simulink model "VDSE_2019b1"  (R2022b)
settings: Solver=ode5  StartTime=0.0  StopTime=T_simulation  FixedStep=simulation_step_time  RelTol=1e-3
values from neighbouring files (symbols this model uses):
  A = 2    [vehicle_parameters_script.m]
  bump_height = 0    [vehicle_parameters_script.m]
  bump_length = 0    [vehicle_parameters_script.m]
  bump_time = 0    [vehicle_parameters_script.m]
  cd = 0.35    [vehicle_parameters_script.m]
  cF = 5000    [vehicle_parameters_script.m]
  clF = -0.15    [vehicle_parameters_script.m]
  clR = -0.20    (= -0.2)    [vehicle_parameters_script.m]
  cp_FA = 30    [vehicle_parameters_script.m]
  cp_RA = 13    [vehicle_parameters_script.m]
  cR = 5000    [vehicle_parameters_script.m]
  ctF = tireF.VERTICAL_DAMPING    [vehicle_parameters_script.m]
  ctR = tireR.VERTICAL_DAMPING    [vehicle_parameters_script.m]
  enableDriverControl = 1    [vehicle_parameters_script.m]
  enableLongDynamics = 1    [vehicle_parameters_script.m]
  enablePowertrain = 1    [vehicle_parameters_script.m]
  g = 9.806    [vehicle_parameters_script.m]
  Gear_numbers = [1 2 3 4 5 6]    [vehicle_parameters_script.m]
  GR = [2.9 1.8 1.3 1 0.85 0.75]    [vehicle_parameters_script.m]
  hcog = 0.441    [vehicle_parameters_script.m]
  hpc = 0.0    (= 0)    [vehicle_parameters_script.m]
  hrcF = 0.3    [vehicle_parameters_script.m]
  hrcg = (hrcF*lR+hrcR*lF)/(lF+lR)    (= 0.25108)    [vehicle_parameters_script.m]
  hrcR = 0.2    [vehicle_parameters_script.m]
  huFcog = 0.32    [vehicle_parameters_script.m]
  huRcog = 0.32    [vehicle_parameters_script.m]
  i1 = 11.42    [vehicle_parameters_script.m]
  i2 = 3.727    [vehicle_parameters_script.m]
  initial_gear = 1    [vehicle_parameters_script.m]
  JwF = 2.45    [vehicle_parameters_script.m]
  JwR = 2.45    [vehicle_parameters_script.m]
  Jx = 4.12    [vehicle_parameters_script.m]
  Jy = 109.16    [vehicle_parameters_script.m]
  Jz = 105.13    [vehicle_parameters_script.m]
  kF = 40000    [vehicle_parameters_script.m]
  kR = 35000    [vehicle_parameters_script.m]
  kRF = 0    [vehicle_parameters_script.m]
  kRR = 0    [vehicle_parameters_script.m]
  ktF = tireF.VERTICAL_STIFFNESS    [vehicle_parameters_script.m]
  ktR = tireR.VERTICAL_STIFFNESS    [vehicle_parameters_script.m]
  lF = 1.223    [vehicle_parameters_script.m]
  lR = l-lF    (= 1.277)    [vehicle_parameters_script.m]
  m = 340    [vehicle_parameters_script.m]
  max_pressure = 1000    [vehicle_parameters_script.m]
  maxrpm = 4000    [vehicle_parameters_script.m]
  mF = 45    [vehicle_parameters_script.m]
  minrpm = 1500    [vehicle_parameters_script.m]
  mR = 50    [vehicle_parameters_script.m]
  output_samping_time = 0.001    [vehicle_parameters_script.m]
  phi0 = 0    [vehicle_parameters_script.m]
  phi_dot0 = 0    [vehicle_parameters_script.m]
  psi0 = 0    [vehicle_parameters_script.m]
  psi_dot0 = 0    [vehicle_parameters_script.m]
  RearRatio = 1    [vehicle_parameters_script.m]
  requested_speed = 120/3.6    (= 33.3333333333)    [vehicle_parameters_script.m]
  rF = tireF.UNLOADED_RADIUS    [vehicle_parameters_script.m]
  rho = 1.2    [vehicle_parameters_script.m]
  rR = tireR.UNLOADED_RADIUS    [vehicle_parameters_script.m]
  steer_ratio = 13.25    [vehicle_parameters_script.m]
  TFL = 0    [vehicle_parameters_script.m]
  TFR = 0    [vehicle_parameters_script.m]
  theta0 = 0    [vehicle_parameters_script.m]
  theta_dot0 = 0    [vehicle_parameters_script.m]
  TRL = 0    [vehicle_parameters_script.m]
  TRR = 0    [vehicle_parameters_script.m]
  Vx0 = 0.01/3.6    (= 0.00277777777778)    [vehicle_parameters_script.m]
  Vy0 = 0    [vehicle_parameters_script.m]
  Vz0 = 0    [vehicle_parameters_script.m]
  wF = 1.578    [vehicle_parameters_script.m]
  wR = 1.544    [vehicle_parameters_script.m]
  x0 = 0    [vehicle_parameters_script.m]
  xcog_overall = (2*mR*xR+2*xF*mF+m*xs)/(m+2*mF+2*mR)    (= 1.25626415094)    [vehicle_parameters_script.m]
  y0 = 0    [vehicle_parameters_script.m]
  z0 = 0    [vehicle_parameters_script.m]
  zFL0 = 0    [vehicle_parameters_script.m]
  zFL_dot0 = 0    [vehicle_parameters_script.m]
  zFR0 = 0    [vehicle_parameters_script.m]
  zFR_dot0 = 0    [vehicle_parameters_script.m]
  zRL0 = 0    [vehicle_parameters_script.m]
  zRL_dot0 = 0    [vehicle_parameters_script.m]
  zRR0 = 0    [vehicle_parameters_script.m]
  zRR_dot0 = 0    [vehicle_parameters_script.m]
undefined symbols (not defined in the file or in its folder): Bxf, Bxr, Byf, Byr, Cxf, Cxr, Cyf, Cyr, DiscIntNeverNeededParam, Dxf, Dxr, Dyf, Dyr, exf, exr, eyf, eyr, FNOMINf, FNOMINr, Ldwf, Ldwr, PCX1f, PCX1r, PCY1f, PCY1r, PDX1f, PDX1r, PDX2f, PDX2r, PDY1f, PDY1r, PDY2f, PDY2r, PDY3f, PDY3r, PEX1f, PEX1r, PEX2f, PEX2r, PEX3f, PEX3r, PEX4f, PEX4r, PEY1f, PEY1r, PEY2f, PEY2r, PEY3f, PEY3r, PEY4f, PEY4r, PHX1f, PHX1r, PHX2f, PHX2r, PHY1f, PHY1r, PHY2f, PHY2r, PHY3f ... (+147)
libraries: simulink x55, mfeval_LIB x4, slpidlib x1
(part 4 of 7)

== system VDSE_2019b1/14-DOF VEHICLE MODEL/SUSPENSION/FRONT SUSPENSION/SUSPENSION FL ==
  z [m] : Inport
  Vz [m/s] : Inport  Port=2
  phi [rad] : Inport  Port=3
  phi_dot [rad/s] : Inport  Port=4
  theta [rad] : Inport  Port=5
  theta_dot [rad/s] : Inport  Port=6
  zFR [m] : Inport  Port=7
  yFL_road [m] : Inport  Port=8
  FL : Subsystem
  TIRE VERTICAL DEFLECTION : Subsystem
  fFLz [N] : Outport
  zFL_dot [m/s] : Outport  Port=2
  zFL [m] : Outport  Port=3
  wires:
  FL/2(zFL_dot [m/s]) -> TIRE VERTICAL DEFLECTION/2(zFL_dot [m/s]), zFL_dot [m/s]/1
  z [m]/1 -> FL/1(z [m])
  TIRE VERTICAL DEFLECTION/1(fFLz [N]) -> fFLz [N]/1
  theta [rad]/1 -> FL/5(theta [rad])
  zFR [m]/1 -> FL/7(zFR [m])
  Vz [m/s]/1 -> FL/2(Vz [m/s])
  yFL_road [m]/1 -> TIRE VERTICAL DEFLECTION/3(yFL_road [m]), FL/8(yFL_road [m])
  phi_dot [rad/s]/1 -> FL/4(phi_dot [rad/s])
  FL/1(zFL [m]) -> TIRE VERTICAL DEFLECTION/1(zFL [m]), zFL [m]/1
  phi [rad]/1 -> FL/3(phi [rad])
  theta_dot [rad/s]/1 -> FL/6(theta_dot [rad/s])

== system VDSE_2019b1/14-DOF VEHICLE MODEL/SUSPENSION/FRONT SUSPENSION/SUSPENSION FR ==
  z [m] : Inport
  Vz [m/s] : Inport  Port=2
  phi [rad] : Inport  Port=3
  phi_dot [rad/s] : Inport  Port=4
  theta [rad] : Inport  Port=5
  theta_dot [rad/s] : Inport  Port=6
  zFL [m] : Inport  Port=7
  yFR_road [m] : Inport  Port=8
  FR : Subsystem
  TIRE VERTICAL DEFLECTION : Subsystem
  fFRz [N] : Outport
  zFR [m] : Outport  Port=2
  zFR_dot [m/s] : Outport  Port=3
  wires:
  FR/2(zFR_dot [m/s]) -> zFR_dot [m/s]/1, TIRE VERTICAL DEFLECTION/2(zFR_dot [m/s])
  yFR_road [m]/1 -> FR/8(yFR_road [m]), TIRE VERTICAL DEFLECTION/3(yFR_road [m])
  z [m]/1 -> FR/1(z [m])
  TIRE VERTICAL DEFLECTION/1(fFRz [N]) -> fFRz [N]/1
  theta [rad]/1 -> FR/5(theta [rad])
  zFL [m]/1 -> FR/7(zFL [m])
  Vz [m/s]/1 -> FR/2(Vz [m/s])
  phi_dot [rad/s]/1 -> FR/4(phi_dot [rad/s])
  FR/1(zFR [m]) -> TIRE VERTICAL DEFLECTION/1(zFR [m]), zFR [m]/1
  phi [rad]/1 -> FR/3(phi [rad])
  theta_dot [rad/s]/1 -> FR/6(theta_dot [rad/s])

== system VDSE_2019b1/14-DOF VEHICLE MODEL/SUSPENSION/Load Transfer/Coupling of load transfer and suspension reaction ==
  Longidutinal Load Transfer [N] : Inport
  Lateral Load Transfer - Front [N] : Inport  Port=2
  Lateral Load Transfer - Rear [N] : Inport  Port=3
  <fFLz [N]> : Inport  Port=4
  <fFRz [N]> : Inport  Port=5
  <fRLz [N]> : Inport  Port=6
  <fRRz [N]> : Inport  Port=7
  Add{,1..4} (5 alike) : Sum
  Add5 : Sum  Inputs=+-
  Add6 : Sum  Inputs=-+
  Add7 : Sum  Inputs=--
  Lateral Load Transfer - Front [N]1 : InportShadow  Port=2
  Lateral Load Transfer - Rear [N]1 : InportShadow  Port=3
  Longidutinal Load Transfer [N]1 : InportShadow
  Longidutinal Load Transfer [N]2 : InportShadow
  Longidutinal Load Transfer [N]3 : InportShadow
  FLz_Overall [N] : Outport
  FRz_Overall [N] : Outport  Port=2
  RLz_Overall [N] : Outport  Port=3
  RRz_Overall [N] : Outport  Port=4
  wires:
  <fFRz [N]>/1 -> Add1/2
  Lateral Load Transfer - Rear [N]/1 -> Add5/2
  Longidutinal Load Transfer [N]/1 -> Add7/1
  Add7/1 -> Add/1  "FL Dynamic LT"
  Lateral Load Transfer - Front [N]/1 -> Add7/2
  Add4/1 -> Add3/1  "RR Dynamic LT"
  Add6/1 -> Add1/1  "FR Dynamic LT"
  Add5/1 -> Add2/1  "RL Dynamic LT"
  <fRRz [N]>/1 -> Add3/2
  <fFLz [N]>/1 -> Add/2
  <fRLz [N]>/1 -> Add2/2
  Add1/1 -> FRz_Overall [N]/1  "FRz_Overall [N]"
  Add3/1 -> RRz_Overall [N]/1  "RRz_Overall [N]"
  Add/1 -> FLz_Overall [N]/1  "FLz_Overall [N]"
  Add2/1 -> RLz_Overall [N]/1  "RLz_Overall [N]"
  Longidutinal Load Transfer [N]1/1 -> Add6/1
  Longidutinal Load Transfer [N]2/1 -> Add5/1
  Longidutinal Load Transfer [N]3/1 -> Add4/1
  Lateral Load Transfer - Front [N]1/1 -> Add6/2
  Lateral Load Transfer - Rear [N]1/1 -> Add4/2

== system VDSE_2019b1/14-DOF VEHICLE MODEL/SUSPENSION/Load Transfer/Dynamic Lateral Load Transfer - Front ==
  ay [m/s^2] : Inport
  Add : Sum
  Gain : Gain  Gain=lR/(lR+lF)
  Gain1 : Gain  Gain=2*mF*huFcog/wF
  Gain2 : Gain  Gain=m*hrcF/wF
  Lat. Dynamic Transfer [N] : Outport
  wires:
  ay [m/s^2]/1 -> Gain2/1, Gain1/1
  Gain2/1 -> Gain/1
  Add/1 -> Lat. Dynamic Transfer [N]/1
  Gain1/1 -> Add/2
  Gain/1 -> Add/1

== system VDSE_2019b1/14-DOF VEHICLE MODEL/SUSPENSION/Load Transfer/Dynamic Lateral Load Transfer - Rear ==
  ay [m/s^2] : Inport
  Add : Sum
  Gain : Gain  Gain=lF/(lR+lF)
  Gain1 : Gain  Gain=2*mR*huRcog/wR
  Gain2 : Gain  Gain=m*hrcR/wR
  Lat. Dynamic Transfer [N] : Outport
  wires:
  Add/1 -> Lat. Dynamic Transfer [N]/1
  Gain1/1 -> Add/2
  ay [m/s^2]/1 -> Gain2/1, Gain1/1
  Gain2/1 -> Gain/1
  Gain/1 -> Add/1

== system VDSE_2019b1/14-DOF VEHICLE MODEL/SUSPENSION/Load Transfer/Dynamic Longitudinal Load Transfer ==
  ax [m/s^2] : Inport
  Add : Sum
  Gain : Gain  Gain=1/2*hpc*m/(lF+lR)/2
  Gain1 : Gain  Gain=(mF*huFcog + mR*huRcog)/(lF+lR)
  Long. Dynamic Transfer [N] : Outport
  wires:
  ax [m/s^2]/1 -> Gain1/1, Gain/1
  Gain/1 -> Add/1
  Add/1 -> Long. Dynamic Transfer [N]/1
  Gain1/1 -> Add/2

== system VDSE_2019b1/14-DOF VEHICLE MODEL/SUSPENSION/REAR SUSPENSION/SUSPENSION RL ==
  z [m] : Inport
  Vz [m/s] : Inport  Port=2
  phi [rad] : Inport  Port=3
  phi_dot [rad/s] : Inport  Port=4
  theta [rad] : Inport  Port=5
  theta_dot [rad/s] : Inport  Port=6
  zRR [m] : Inport  Port=7
  yRL_road [m] : Inport  Port=8
  RL : Subsystem
  TIRE VERTICAL DEFLECTION : Subsystem
  fRLz [N] : Outport
  zRL_dot [m/s] : Outport  Port=2
  zRL [m] : Outport  Port=3
  wires:
  RL/2(zRL_dot [m/s]) -> TIRE VERTICAL DEFLECTION/2(zRL_dot [m/s]), zRL_dot [m/s]/1
  z [m]/1 -> RL/1(z [m])
  TIRE VERTICAL DEFLECTION/1(fRLz [N]) -> fRLz [N]/1  "fRLz [N]"
  theta [rad]/1 -> RL/5(theta [rad])
  zRR [m]/1 -> RL/7(zRR [m])
  Vz [m/s]/1 -> RL/2(Vz [m/s])
  yRL_road [m]/1 -> TIRE VERTICAL DEFLECTION/3(yRL_road [m]), RL/8(yRL_road [m])
  phi_dot [rad/s]/1 -> RL/4(phi_dot [rad/s])
  RL/1(zRL [m]) -> TIRE VERTICAL DEFLECTION/1(zRL [m]), zRL [m]/1
  phi [rad]/1 -> RL/3(phi [rad])
  theta_dot [rad/s]/1 -> RL/6(theta_dot [rad/s])

== system VDSE_2019b1/14-DOF VEHICLE MODEL/SUSPENSION/REAR SUSPENSION/SUSPENSION RR ==
  z [m] : Inport
  Vz [m/s] : Inport  Port=2
  phi [rad] : Inport  Port=3
  phi_dot [rad/s] : Inport  Port=4
  theta [rad] : Inport  Port=5
  theta_dot [rad/s] : Inport  Port=6
  zRL [m] : Inport  Port=7
  yRR_road [m] : Inport  Port=8
  RR : Subsystem
  TIRE VERTICAL DEFLECTION : Subsystem
  fRRz [N] : Outport
  zRR [m] : Outport  Port=2
  zRR_dot [m/s] : Outport  Port=3
  wires:
  RR/2(zRR_dot [m/s]) -> TIRE VERTICAL DEFLECTION/2(zRR_dot [m/s]), zRR_dot [m/s]/1
  yRR_road [m]/1 -> TIRE VERTICAL DEFLECTION/3(yRR_road [m]), RR/8(yRR_road [m])
  z [m]/1 -> RR/1(z [m])
  TIRE VERTICAL DEFLECTION/1(fRRz [N]) -> fRRz [N]/1
  theta [rad]/1 -> RR/5(theta [rad])
  zRL [m]/1 -> RR/7(zRL [m])
  Vz [m/s]/1 -> RR/2(Vz [m/s])
  phi_dot [rad/s]/1 -> RR/4(phi_dot [rad/s])
  RR/1(zRR [m]) -> TIRE VERTICAL DEFLECTION/1(zRR [m]), zRR [m]/1
  phi [rad]/1 -> RR/3(phi [rad])
  theta_dot [rad/s]/1 -> RR/6(theta_dot [rad/s])

== system VDSE_2019b1/14-DOF VEHICLE MODEL/WHEEL ASSEMBLY/WHEEL ASSEMBLY BCD/SIDE SLIP ANGLE CALCULATION ==
  Vx [m/s] : Inport
  Vy [m/s] : Inport  Port=2
  Add : Sum
  Atan2 : Trigonometry  Operator=atan2
  Clock : Clock
  Constant : Constant  Value=enableLongDynamics
  Constant1 : Constant  Value=Vx0
  Constant2 : Constant  Value=0
  Sqrt : Sqrt
  Square : Math  Operator=square
  Square1 : Math  Operator=square
  Switch : Switch  Criteria=u2 > Threshold  SaturateOnIntegerOverflow=off  InputSameDT=off
  Switch1 : Switch  Criteria=u2 > Threshold  Threshold=0.01  SaturateOnIntegerOverflow=off  InputSameDT=off
  Vy [m/s]1 : InportShadow  Port=2
  V [m/s] : Outport
  beta [rad] : Outport  Port=2
  wires:
  Clock/1 -> Switch1/2
  Constant2/1 -> Switch1/3
  Switch1/1 -> Switch/2
  Constant1/1 -> Switch/3
  Constant/1 -> Switch1/1
  Switch/1 -> Atan2/2, Square/1
  Square1/1 -> Add/2
  Square/1 -> Add/1
  Vy [m/s]/1 -> Square1/1
  Vx [m/s]/1 -> Switch/1
  Add/1 -> Sqrt/1
  Sqrt/1 -> V [m/s]/1
  Atan2/1 -> beta [rad]/1
  Vy [m/s]1/1 -> Atan2/1

== system VDSE_2019b1/14-DOF VEHICLE MODEL/WHEEL ASSEMBLY/WHEEL ASSEMBLY BCD/TIRE PARAMETERS ==
  Constant : Constant  Value=Bxf
  Constant1 : Constant  Value=Cxf
  Constant10 : Constant  Value=Cyr
  Constant11 : Constant  Value=Dyr
  Constant2 : Constant  Value=Dxf
  Constant3 : Constant  Value=Bxr
  Constant4 : Constant  Value=Cxr
  Constant5 : Constant  Value=Dxr
  Constant6 : Constant  Value=Byf
  Constant7 : Constant  Value=Cyf
  Constant8 : Constant  Value=Dyf
  Constant9 : Constant  Value=Byr
  Bxf : Outport
  Cxf : Outport  Port=2
  Dxf : Outport  Port=3
  Bxr : Outport  Port=4
  Cxr : Outport  Port=5
  Dxr : Outport  Port=6
  Byf : Outport  Port=7
  Cyf : Outport  Port=8
  Dyf : Outport  Port=9
  Byr : Outport  Port=10
  Cyr : Outport  Port=11
  Dyr : Outport  Port=12
  wires:
  Constant/1 -> Bxf/1
  Constant1/1 -> Cxf/1
  Constant2/1 -> Dxf/1
  Constant5/1 -> Dxr/1
  Constant4/1 -> Cxr/1
  Constant3/1 -> Bxr/1
  Constant9/1 -> Byr/1
  Constant10/1 -> Cyr/1
  Constant11/1 -> Dyr/1
  Constant8/1 -> Dyf/1
  Constant7/1 -> Cyf/1
  Constant6/1 -> Byf/1

== system VDSE_2019b1/14-DOF VEHICLE MODEL/WHEEL ASSEMBLY/WHEEL ASSEMBLY MFEVAL/SIDE SLIP ANGLE CALCULATION ==
  Vx [m/s] : Inport
  Vy [m/s] : Inport  Port=2
  Add : Sum
  Atan2 : Trigonometry  Operator=atan2
  Clock : Clock
  Constant : Constant  Value=enableLongDynamics
  Constant1 : Constant  Value=Vx0
  Constant2 : Constant  Value=0
  Sqrt : Sqrt
  Square : Math  Operator=square
  Square1 : Math  Operator=square
  Switch : Switch  Criteria=u2 > Threshold  SaturateOnIntegerOverflow=off  InputSameDT=off
  Switch1 : Switch  Criteria=u2 > Threshold  Threshold=0.01  SaturateOnIntegerOverflow=off  InputSameDT=off
  Vy [m/s]1 : InportShadow  Port=2
  V [m/s] : Outport
  beta [rad] : Outport  Port=2
  wires:
  Clock/1 -> Switch1/2
  Constant2/1 -> Switch1/3
  Switch1/1 -> Switch/2
  Constant1/1 -> Switch/3
  Constant/1 -> Switch1/1
  Square1/1 -> Add/2
  Square/1 -> Add/1
  Vy [m/s]/1 -> Square1/1
  Vx [m/s]/1 -> Switch/1
  Add/1 -> Sqrt/1
  Atan2/1 -> beta [rad]/1
  Vy [m/s]1/1 -> Atan2/1
  Switch/1 -> Atan2/2, Square/1
  Sqrt/1 -> V [m/s]/1

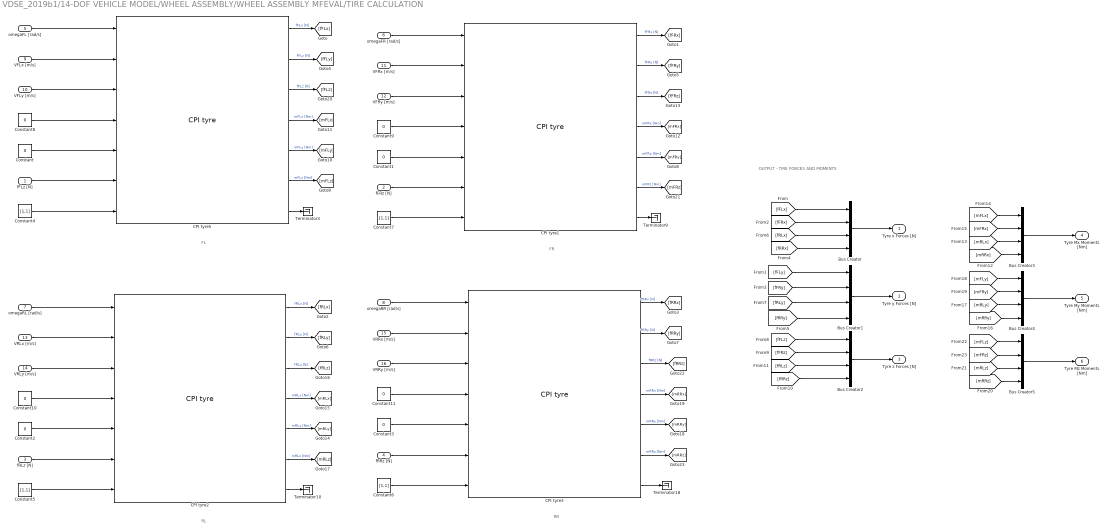
== system VDSE_2019b1/14-DOF VEHICLE MODEL/WHEEL ASSEMBLY/WHEEL ASSEMBLY MFEVAL/TIRE CALCULATION ==
  note: RR
  note: RL
  note: FR
  note: FL
  note: OUTPUT - TIRE FORCES AND MOMENTS
  fFLz [N] : Inport
  fFRz [N] : Inport  Port=2
  fRLz [N] : Inport  Port=3
  fRRz [N] : Inport  Port=4
  omegaFL [rad/s] : Inport  Port=5
  omegaFR [rad/s] : Inport  Port=6
  omegaRL [rad/s] : Inport  Port=7
  omegaRR [rad/s] : Inport  Port=8
  VFLx [m/s] : Inport  Port=9
  VFLy [m/s] : Inport  Port=10
  VFRx [m/s] : Inport  Port=11
  VFRy [m/s] : Inport  Port=12
  VRLx [m/s] : Inport  Port=13
  VRLy [m/s] : Inport  Port=14
  VRRx [m/s] : Inport  Port=15
  VRRy [m/s] : Inport  Port=16
  Bus Creator{,1..5} (6 alike) : BusCreator  Inputs=4
  CPI tyre1 : mfeval_LIB/CPI tyre  Description=Magic Formula 6.1.2 tyre model including relaxation length and transient calculations  userParameterSource=tir_file_front  userSide=2 right  userDynamics=1 steady state  userUseMode=1 combined  enablePressure=off  userPressure=2.3
      settings: SourceProductName=MFeval Library
  CPI tyre2 : mfeval_LIB/CPI tyre  Description=Magic Formula 6.1.2 tyre model including relaxation length and transient calculations  userParameterSource=tir_file_rear  userSide=1 left  userDynamics=1 steady state  userUseMode=1 combined  enablePressure=off  userPressure=2.3
      settings: SourceProductName=MFeval Library
  CPI tyre3 : mfeval_LIB/CPI tyre  Description=Magic Formula 6.1.2 tyre model including relaxation length and transient calculations  userParameterSource=tir_file_rear  userSide=2 right  userDynamics=1 steady state  userUseMode=1 combined  enablePressure=off  userPressure=2.3
      settings: SourceProductName=MFeval Library
  CPI tyre5 : mfeval_LIB/CPI tyre  Description=Magic Formula 6.1.2 tyre model including relaxation length and transient calculations  userParameterSource=tir_file_front  userSide=1 left  userDynamics=1 steady state  userUseMode=1 combined  enablePressure=off  userPressure=2.3
      settings: SourceProductName=MFeval Library
  Constant{,1..3,8..11} (8 alike) : Constant  Value=0
  Constant{4..7} (4 alike) : Constant  Value=[1,1]
  Terminator{3,9..10,18} (4 alike) : Terminator
  Tyre x Forces [N] : Outport
  Tyre y Forces [N] : Outport  Port=2
  Tyre z Forces [N] : Outport  Port=3
  Tyre Mx Moments [Nm] : Outport  Port=4
  Tyre My Moments [Nm] : Outport  Port=5
  Tyre Mz Moments [Nm] : Outport  Port=6
  wires:
  Constant11/1 -> CPI tyre3/4
  Constant10/1 -> CPI tyre2/4
  Constant9/1 -> CPI tyre1/4
  Constant8/1 -> CPI tyre5/4
  CPI tyre3/3 -> [fRRz]  "fRRz [N]"
  CPI tyre3/6 -> [mRRz]  "mRRz [Nm]"
  CPI tyre3/4 -> [mRRx]  "mRRx [Nm]"
  CPI tyre3/5 -> [mRRy]  "mRRy [Nm]"
  CPI tyre2/3 -> [fRLz]  "fRLz [N]"
  CPI tyre2/6 -> [mRLz]  "mRLz [Nm]"
  CPI tyre2/4 -> [mRLx]  "mRLx [Nm]"
  CPI tyre2/5 -> [mRLy]  "mRLy [Nm]"
  CPI tyre1/3 -> [fFRz]  "fFRz [N]"
  CPI tyre1/6 -> [mFRz]  "mFRz [Nm]"
  CPI tyre1/4 -> [mFRx]  "mFRx [Nm]"
  CPI tyre1/5 -> [mFRy]  "mFRy [Nm]"
  CPI tyre5/3 -> [fFLz]  "fFLz [N]"
  CPI tyre5/4 -> [mFLx]  "mFLx [Nm]"
  CPI tyre5/5 -> [mFLy]  "mFLy [Nm]"
  Bus Creator5/1 -> Tyre Mz Moments [Nm]/1
  [mFRz] -> Bus Creator5/2
  [mRLz] -> Bus Creator5/3
  [mRRz] -> Bus Creator5/4
  [mFLz] -> Bus Creator5/1
  [mFLy] -> Bus Creator4/1
  [mRRy] -> Bus Creator4/4
  [mRLy] -> Bus Creator4/3
  [mFRy] -> Bus Creator4/2
  Bus Creator4/1 -> Tyre My Moments [Nm]/1
  Bus Creator3/1 -> Tyre Mx Moments [Nm]/1
  [mFRx] -> Bus Creator3/2
  [mRLx] -> Bus Creator3/3
  [mRRx] -> Bus Creator3/4
  [mFLx] -> Bus Creator3/1
  [fFLz] -> Bus Creator2/1
  [fRRz] -> Bus Creator2/4
  [fRLz] -> Bus Creator2/3
  [fFRz] -> Bus Creator2/2
  Bus Creator2/1 -> Tyre z Forces [N]/1
  Bus Creator1/1 -> Tyre y Forces [N]/1
  Bus Creator/1 -> Tyre x Forces [N]/1
  [fFRy] -> Bus Creator1/2
  [fRLy] -> Bus Creator1/3
  [fRRy] -> Bus Creator1/4
  [fFLy] -> Bus Creator1/1
  [fRRx] -> Bus Creator/4
  [fRLx] -> Bus Creator/3
  [fFRx] -> Bus Creator/2
  [fFLx] -> Bus Creator/1
  CPI tyre3/2 -> [fRRy]  "fRRy [N]"
  CPI tyre2/2 -> [fRLy]  "fRLy [N]"
  CPI tyre1/2 -> [fFRy]  "fFRy [N]"
  CPI tyre5/2 -> [fFLy]  "fFLy [N]"
  CPI tyre2/1 -> [fRLx]  "fRLx [N]"
  CPI tyre3/1 -> [fRRx]  "fRRx [N]"
  CPI tyre1/1 -> [fFRx]  "fFRx [N]"
  CPI tyre5/1 -> [fFLx]  "fFLx [N]"
  CPI tyre3/7 -> Terminator18/1
  CPI tyre2/7 -> Terminator10/1
  CPI tyre1/7 -> Terminator9/1
  CPI tyre5/7 -> Terminator3/1
  CPI tyre5/6 -> [mFLz]  "mFLz [Nm]"
  VRRx [m/s]/1 -> CPI tyre3/2
  VRRy [m/s]/1 -> CPI tyre3/3
  VRLy [m/s]/1 -> CPI tyre2/3
  VRLx [m/s]/1 -> CPI tyre2/2
  VFRy [m/s]/1 -> CPI tyre1/3
  VFRx [m/s]/1 -> CPI tyre1/2
  VFLx [m/s]/1 -> CPI tyre5/2
  VFLy [m/s]/1 -> CPI tyre5/3
  omegaRR [rad/s]/1 -> CPI tyre3/1
  omegaRL [rad/s]/1 -> CPI tyre2/1
  omegaFR [rad/s]/1 -> CPI tyre1/1
  omegaFL [rad/s]/1 -> CPI tyre5/1
  Constant7/1 -> CPI tyre1/7
  Constant6/1 -> CPI tyre3/7
  Constant5/1 -> CPI tyre2/7
  Constant4/1 -> CPI tyre5/7
  Constant3/1 -> CPI tyre3/5
  Constant2/1 -> CPI tyre2/5
  Constant1/1 -> CPI tyre1/5
  Constant/1 -> CPI tyre5/5
  fFLz [N]/1 -> CPI tyre5/6
  fRLz [N]/1 -> CPI tyre2/6
  fRRz [N]/1 -> CPI tyre3/6
  fFRz [N]/1 -> CPI tyre1/6

== system VDSE_2019b1/14-DOF VEHICLE MODEL/WHEEL ASSEMBLY/WHEEL ASSEMBLY PACEIJKA/SIDE SLIP ANGLE CALCULATION ==
  Vx [m/s] : Inport
  Vy [m/s] : Inport  Port=2
  Add : Sum
  Atan2 : Trigonometry  Operator=atan2
  Clock : Clock
  Constant : Constant  Value=enableLongDynamics
  Constant1 : Constant  Value=Vx0
  Constant2 : Constant  Value=0
  Sqrt : Sqrt
  Square : Math  Operator=square
  Square1 : Math  Operator=square
  Switch : Switch  Criteria=u2 > Threshold  SaturateOnIntegerOverflow=off  InputSameDT=off
  Switch1 : Switch  Criteria=u2 > Threshold  Threshold=0.01  SaturateOnIntegerOverflow=off  InputSameDT=off
  Vy [m/s]1 : InportShadow  Port=2
  V [m/s] : Outport
  beta [rad] : Outport  Port=2
  wires:
  Vy [m/s]1/1 -> Atan2/1
  Atan2/1 -> beta [rad]/1
  Sqrt/1 -> V [m/s]/1
  Add/1 -> Sqrt/1
  Vx [m/s]/1 -> Switch/1
  Vy [m/s]/1 -> Square1/1
  Square/1 -> Add/1
  Square1/1 -> Add/2
  Switch/1 -> Atan2/2, Square/1
  Constant/1 -> Switch1/1
  Constant1/1 -> Switch/3
  Switch1/1 -> Switch/2
  Constant2/1 -> Switch1/3
  Clock/1 -> Switch1/2

== system VDSE_2019b1/14-DOF VEHICLE MODEL/WHEEL ASSEMBLY/WHEEL ASSEMBLY PACEIJKA/TIRE PARAMETERS ==
  Mux1 : Mux  Inputs=91
  Mux2 : Mux  Inputs=91
  TIRE PARAMETERS - FRONT AXLE : Subsystem
  TIRE PARAMETERS - REAR AXLE : Subsystem
  Tire Parameters Front Axle : Outport
  Tire Parameters Rear Axle : Outport  Port=2
  wires:
  TIRE PARAMETERS - FRONT AXLE/29(PCY1) -> Mux1/29
  TIRE PARAMETERS - FRONT AXLE/18(PKY3) -> Mux1/18
  TIRE PARAMETERS - FRONT AXLE/1(PHX1) -> Mux1/1
  TIRE PARAMETERS - FRONT AXLE/48(RVY4) -> Mux1/48
  TIRE PARAMETERS - FRONT AXLE/41(RBY1) -> Mux1/41
  TIRE PARAMETERS - FRONT AXLE/8(PEX3) -> Mux1/8
  TIRE PARAMETERS - FRONT AXLE/23(PHY1) -> Mux1/23
  TIRE PARAMETERS - FRONT AXLE/46(RVY2) -> Mux1/46
  TIRE PARAMETERS - FRONT AXLE/5(PCX1) -> Mux1/5
  TIRE PARAMETERS - FRONT AXLE/19(PVY1) -> Mux1/19
  TIRE PARAMETERS - FRONT AXLE/22(PVY4) -> Mux1/22
  TIRE PARAMETERS - FRONT AXLE/53(RHY1) -> Mux1/53
  TIRE PARAMETERS - FRONT AXLE/7(PEX2) -> Mux1/7
  TIRE PARAMETERS - FRONT AXLE/37(RCX1) -> Mux1/37
  TIRE PARAMETERS - FRONT AXLE/51(REY1) -> Mux1/51
  TIRE PARAMETERS - FRONT AXLE/28(PDY3) -> Mux1/28
  TIRE PARAMETERS - FRONT AXLE/36(RBX2) -> Mux1/36
  TIRE PARAMETERS - FRONT AXLE/34(ey) -> Mux1/34
  TIRE PARAMETERS - FRONT AXLE/10(PKX1) -> Mux1/10
  TIRE PARAMETERS - FRONT AXLE/30(PEY1) -> Mux1/30
  TIRE PARAMETERS - FRONT AXLE/17(PKY2) -> Mux1/17
  TIRE PARAMETERS - FRONT AXLE/2(PHX2) -> Mux1/2
  TIRE PARAMETERS - FRONT AXLE/33(PEY4) -> Mux1/33
  TIRE PARAMETERS - FRONT AXLE/39(REX2) -> Mux1/39
  TIRE PARAMETERS - FRONT AXLE/45(RVY1) -> Mux1/45
  TIRE PARAMETERS - FRONT AXLE/52(REY2) -> Mux1/52
  TIRE PARAMETERS - FRONT AXLE/21(PVY3) -> Mux1/21
  TIRE PARAMETERS - FRONT AXLE/3(PDX1) -> Mux1/3
  TIRE PARAMETERS - FRONT AXLE/6(PEX1) -> Mux1/6
  TIRE PARAMETERS - FRONT AXLE/4(PDX2) -> Mux1/4
  TIRE PARAMETERS - FRONT AXLE/49(RVY5) -> Mux1/49
  TIRE PARAMETERS - FRONT AXLE/44(RCY1) -> Mux1/44
  TIRE PARAMETERS - FRONT AXLE/25(PHY3) -> Mux1/25
  TIRE PARAMETERS - FRONT AXLE/24(PHY2) -> Mux1/24
  TIRE PARAMETERS - FRONT AXLE/54(RHY2) -> Mux1/54
  TIRE PARAMETERS - FRONT AXLE/43(RBY3) -> Mux1/43
  TIRE PARAMETERS - FRONT AXLE/13(ex) -> Mux1/13
  TIRE PARAMETERS - FRONT AXLE/31(PEY2) -> Mux1/31
  TIRE PARAMETERS - FRONT AXLE/14(PVX1) -> Mux1/14
  TIRE PARAMETERS - FRONT AXLE/35(RBX1) -> Mux1/35
  TIRE PARAMETERS - FRONT AXLE/15(PVX2) -> Mux1/15
  TIRE PARAMETERS - FRONT AXLE/27(PDY2) -> Mux1/27
  TIRE PARAMETERS - FRONT AXLE/20(PVY2) -> Mux1/20
  TIRE PARAMETERS - FRONT AXLE/11(PKX2) -> Mux1/11
  TIRE PARAMETERS - FRONT AXLE/50(RVY6) -> Mux1/50
  TIRE PARAMETERS - FRONT AXLE/32(PEY3) -> Mux1/32
  Mux1/1 -> Tire Parameters Front Axle/1
  TIRE PARAMETERS - FRONT AXLE/47(RVY3) -> Mux1/47
  TIRE PARAMETERS - FRONT AXLE/9(PEX4) -> Mux1/9
  TIRE PARAMETERS - FRONT AXLE/40(RHX1) -> Mux1/40
  TIRE PARAMETERS - FRONT AXLE/38(REX1) -> Mux1/38
  TIRE PARAMETERS - FRONT AXLE/42(RBY2) -> Mux1/42
  TIRE PARAMETERS - FRONT AXLE/26(PDY1) -> Mux1/26
  TIRE PARAMETERS - FRONT AXLE/12(PKX3) -> Mux1/12
  TIRE PARAMETERS - FRONT AXLE/16(PKY1) -> Mux1/16
  TIRE PARAMETERS - REAR AXLE/16(PKY1) -> Mux2/16
  TIRE PARAMETERS - REAR AXLE/12(PKX3) -> Mux2/12
  TIRE PARAMETERS - REAR AXLE/26(PDY1) -> Mux2/26
  TIRE PARAMETERS - REAR AXLE/42(RBY2) -> Mux2/42
  TIRE PARAMETERS - REAR AXLE/38(REX1) -> Mux2/38
  TIRE PARAMETERS - REAR AXLE/40(RHX1) -> Mux2/40
  TIRE PARAMETERS - REAR AXLE/9(PEX4) -> Mux2/9
  TIRE PARAMETERS - REAR AXLE/47(RVY3) -> Mux2/47
  Mux2/1 -> Tire Parameters Rear Axle/1
  TIRE PARAMETERS - REAR AXLE/32(PEY3) -> Mux2/32
  TIRE PARAMETERS - REAR AXLE/50(RVY6) -> Mux2/50
  TIRE PARAMETERS - REAR AXLE/11(PKX2) -> Mux2/11
  TIRE PARAMETERS - REAR AXLE/20(PVY2) -> Mux2/20
  TIRE PARAMETERS - REAR AXLE/27(PDY2) -> Mux2/27
  TIRE PARAMETERS - REAR AXLE/15(PVX2) -> Mux2/15
  TIRE PARAMETERS - REAR AXLE/35(RBX1) -> Mux2/35
  TIRE PARAMETERS - REAR AXLE/14(PVX1) -> Mux2/14
  TIRE PARAMETERS - REAR AXLE/31(PEY2) -> Mux2/31
  TIRE PARAMETERS - REAR AXLE/13(ex) -> Mux2/13
  TIRE PARAMETERS - REAR AXLE/43(RBY3) -> Mux2/43
  TIRE PARAMETERS - REAR AXLE/54(RHY2) -> Mux2/54
  TIRE PARAMETERS - REAR AXLE/24(PHY2) -> Mux2/24
  TIRE PARAMETERS - REAR AXLE/25(PHY3) -> Mux2/25
  TIRE PARAMETERS - REAR AXLE/44(RCY1) -> Mux2/44
  TIRE PARAMETERS - REAR AXLE/49(RVY5) -> Mux2/49
  TIRE PARAMETERS - REAR AXLE/4(PDX2) -> Mux2/4
  TIRE PARAMETERS - REAR AXLE/6(PEX1) -> Mux2/6
  TIRE PARAMETERS - REAR AXLE/3(PDX1) -> Mux2/3
  TIRE PARAMETERS - REAR AXLE/21(PVY3) -> Mux2/21
  TIRE PARAMETERS - REAR AXLE/52(REY2) -> Mux2/52
  TIRE PARAMETERS - REAR AXLE/45(RVY1) -> Mux2/45
  TIRE PARAMETERS - REAR AXLE/39(REX2) -> Mux2/39
  TIRE PARAMETERS - REAR AXLE/33(PEY4) -> Mux2/33
  TIRE PARAMETERS - REAR AXLE/2(PHX2) -> Mux2/2
  TIRE PARAMETERS - REAR AXLE/17(PKY2) -> Mux2/17
  TIRE PARAMETERS - REAR AXLE/30(PEY1) -> Mux2/30
  TIRE PARAMETERS - REAR AXLE/10(PKX1) -> Mux2/10
  TIRE PARAMETERS - REAR AXLE/34(ey) -> Mux2/34
  TIRE PARAMETERS - REAR AXLE/36(RBX2) -> Mux2/36
  TIRE PARAMETERS - REAR AXLE/28(PDY3) -> Mux2/28
  TIRE PARAMETERS - REAR AXLE/51(REY1) -> Mux2/51
  TIRE PARAMETERS - REAR AXLE/37(RCX1) -> Mux2/37
  TIRE PARAMETERS - REAR AXLE/7(PEX2) -> Mux2/7
  TIRE PARAMETERS - REAR AXLE/53(RHY1) -> Mux2/53
  TIRE PARAMETERS - REAR AXLE/22(PVY4) -> Mux2/22
  TIRE PARAMETERS - REAR AXLE/19(PVY1) -> Mux2/19
  TIRE PARAMETERS - REAR AXLE/5(PCX1) -> Mux2/5
  TIRE PARAMETERS - REAR AXLE/46(RVY2) -> Mux2/46
  TIRE PARAMETERS - REAR AXLE/23(PHY1) -> Mux2/23
  TIRE PARAMETERS - REAR AXLE/8(PEX3) -> Mux2/8
  TIRE PARAMETERS - REAR AXLE/41(RBY1) -> Mux2/41
  TIRE PARAMETERS - REAR AXLE/48(RVY4) -> Mux2/48
  TIRE PARAMETERS - REAR AXLE/1(PHX1) -> Mux2/1
  TIRE PARAMETERS - REAR AXLE/18(PKY3) -> Mux2/18
  TIRE PARAMETERS - REAR AXLE/29(PCY1) -> Mux2/29
  TIRE PARAMETERS - REAR AXLE/55(FNOMIN) -> Mux2/55
  TIRE PARAMETERS - FRONT AXLE/55(FNOMIN) -> Mux1/55
  TIRE PARAMETERS - FRONT AXLE/56(QHZ1) -> Mux1/56
  TIRE PARAMETERS - FRONT AXLE/57(QHZ2) -> Mux1/57
  TIRE PARAMETERS - FRONT AXLE/58(QHZ3) -> Mux1/58
  TIRE PARAMETERS - FRONT AXLE/59(QHZ4) -> Mux1/59
  TIRE PARAMETERS - FRONT AXLE/60(QBZ1) -> Mux1/60
  TIRE PARAMETERS - FRONT AXLE/61(QBZ2) -> Mux1/61
  TIRE PARAMETERS - FRONT AXLE/62(QBZ3) -> Mux1/62
  TIRE PARAMETERS - FRONT AXLE/63(QBZ4) -> Mux1/63
  TIRE PARAMETERS - FRONT AXLE/64(QBZ5) -> Mux1/64
  TIRE PARAMETERS - FRONT AXLE/65(QCZ1) -> Mux1/65
  TIRE PARAMETERS - FRONT AXLE/66(QDZ1) -> Mux1/66
  TIRE PARAMETERS - FRONT AXLE/67(QDZ2) -> Mux1/67
  TIRE PARAMETERS - FRONT AXLE/68(QDZ3) -> Mux1/68
  TIRE PARAMETERS - FRONT AXLE/69(QDZ4) -> Mux1/69
  TIRE PARAMETERS - FRONT AXLE/70(QEZ1) -> Mux1/70
  TIRE PARAMETERS - FRONT AXLE/71(QEZ2) -> Mux1/71
  TIRE PARAMETERS - FRONT AXLE/72(QEZ3) -> Mux1/72
  TIRE PARAMETERS - FRONT AXLE/73(QEZ4) -> Mux1/73
  TIRE PARAMETERS - FRONT AXLE/74(QEZ5) -> Mux1/74
  TIRE PARAMETERS - FRONT AXLE/75(QBZ9) -> Mux1/75
  TIRE PARAMETERS - FRONT AXLE/76(QBZ10) -> Mux1/76
  TIRE PARAMETERS - FRONT AXLE/77(QDZ6) -> Mux1/77
  TIRE PARAMETERS - FRONT AXLE/78(QDZ7) -> Mux1/78
  TIRE PARAMETERS - FRONT AXLE/79(QDZ8) -> Mux1/79
  TIRE PARAMETERS - FRONT AXLE/80(QDZ9) -> Mux1/80
  TIRE PARAMETERS - FRONT AXLE/81(R0) -> Mux1/81
  TIRE PARAMETERS - FRONT AXLE/82(zeta7) -> Mux1/82
  TIRE PARAMETERS - FRONT AXLE/83(SSZ1) -> Mux1/83
  TIRE PARAMETERS - FRONT AXLE/84(SSZ2) -> Mux1/84
  TIRE PARAMETERS - FRONT AXLE/85(SSZ3) -> Mux1/85
  TIRE PARAMETERS - FRONT AXLE/86(SSZ4) -> Mux1/86
  TIRE PARAMETERS - FRONT AXLE/87(QSY1) -> Mux1/87
  TIRE PARAMETERS - FRONT AXLE/88(QSY2) -> Mux1/88
  TIRE PARAMETERS - FRONT AXLE/89(QSY3) -> Mux1/89
  TIRE PARAMETERS - FRONT AXLE/90(QSY4) -> Mux1/90
  TIRE PARAMETERS - FRONT AXLE/91(VREF) -> Mux1/91
  TIRE PARAMETERS - REAR AXLE/56(QHZ1) -> Mux2/56
  TIRE PARAMETERS - REAR AXLE/57(QHZ2) -> Mux2/57
  TIRE PARAMETERS - REAR AXLE/58(QHZ3) -> Mux2/58
  TIRE PARAMETERS - REAR AXLE/59(QHZ4) -> Mux2/59
  TIRE PARAMETERS - REAR AXLE/60(QBZ1) -> Mux2/60
  TIRE PARAMETERS - REAR AXLE/61(QBZ2) -> Mux2/61
  TIRE PARAMETERS - REAR AXLE/62(QBZ3) -> Mux2/62
  TIRE PARAMETERS - REAR AXLE/63(QBZ4) -> Mux2/63
  TIRE PARAMETERS - REAR AXLE/64(QBZ5) -> Mux2/64
  TIRE PARAMETERS - REAR AXLE/65(QCZ1) -> Mux2/65
  TIRE PARAMETERS - REAR AXLE/66(QDZ1) -> Mux2/66
  TIRE PARAMETERS - REAR AXLE/67(QDZ2) -> Mux2/67
  TIRE PARAMETERS - REAR AXLE/68(QDZ3) -> Mux2/68
  TIRE PARAMETERS - REAR AXLE/69(QDZ4) -> Mux2/69
  TIRE PARAMETERS - REAR AXLE/70(QEZ1) -> Mux2/70
  TIRE PARAMETERS - REAR AXLE/71(QEZ2) -> Mux2/71
  TIRE PARAMETERS - REAR AXLE/72(QEZ3) -> Mux2/72
  TIRE PARAMETERS - REAR AXLE/73(QEZ4) -> Mux2/73
  TIRE PARAMETERS - REAR AXLE/74(QEZ5) -> Mux2/74
  TIRE PARAMETERS - REAR AXLE/75(QBZ9) -> Mux2/75
  TIRE PARAMETERS - REAR AXLE/76(QBZ10) -> Mux2/76
  TIRE PARAMETERS - REAR AXLE/77(QDZ6) -> Mux2/77
  TIRE PARAMETERS - REAR AXLE/78(QDZ7) -> Mux2/78
  TIRE PARAMETERS - REAR AXLE/79(QDZ8) -> Mux2/79
  TIRE PARAMETERS - REAR AXLE/80(QDZ9) -> Mux2/80
  TIRE PARAMETERS - REAR AXLE/81(R0) -> Mux2/81
  TIRE PARAMETERS - REAR AXLE/82(zeta7) -> Mux2/82
  TIRE PARAMETERS - REAR AXLE/83(SSZ1) -> Mux2/83
  TIRE PARAMETERS - REAR AXLE/84(SSZ2) -> Mux2/84
  TIRE PARAMETERS - REAR AXLE/85(SSZ3) -> Mux2/85
  TIRE PARAMETERS - REAR AXLE/86(SSZ4) -> Mux2/86
  TIRE PARAMETERS - REAR AXLE/87(QSY1) -> Mux2/87
  TIRE PARAMETERS - REAR AXLE/88(QSY2) -> Mux2/88
  TIRE PARAMETERS - REAR AXLE/89(QSY3) -> Mux2/89
  TIRE PARAMETERS - REAR AXLE/90(QSY4) -> Mux2/90
  TIRE PARAMETERS - REAR AXLE/91(VREF) -> Mux2/91

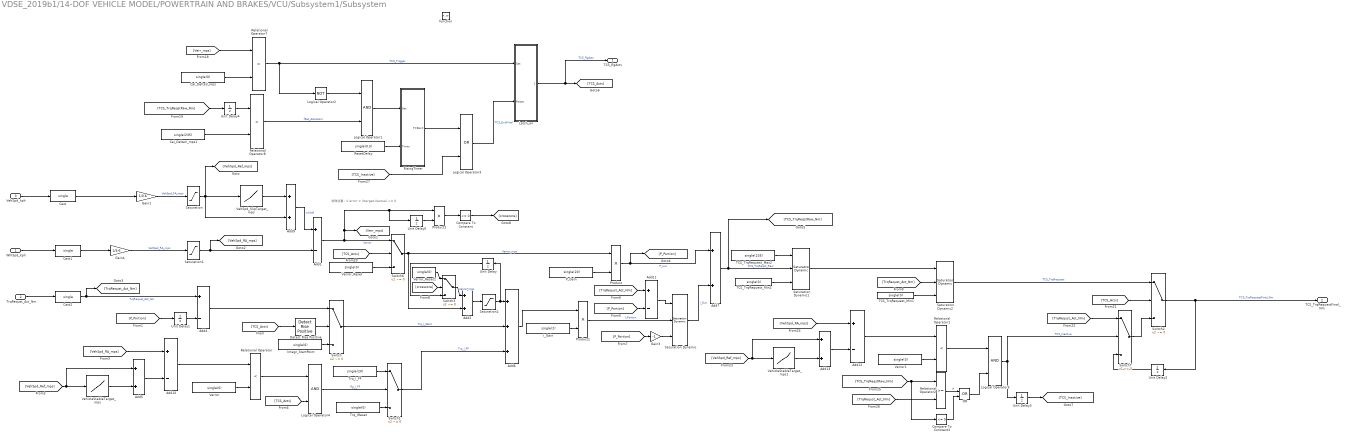
== system VDSE_2019b1/14-DOF VEHICLE MODEL/POWERTRAIN AND BRAKES/VCU/Subsystem1/Subsystem ==
  note: 特殊设置：V error = Vtarget-Vactual <= 0
  WhlSpd_kph : Inport
  TrqRequst_Act_Nm : Inport  Port=2
  VehSpd_kph : Inport  Port=3
  function : TriggerPort  TriggerType=function-call  VariantControl=(inherit)
  Add{1,4,10..12} (5 alike) : Sum  Inputs=+-
  Add{2,5,7,9,13} (5 alike) : Sum
  Add6 : Sum  Inputs=+++
  Cal_DeltaV_mps : Constant  Value=single(0)
  Cal_DeltaV_mps1 : Constant  Value=single(235)
  Cast : DataTypeConversion  OutDataTypeStr=single  SaturateOnIntegerOverflow=off  RndMeth=Floor
  Cast1 : DataTypeConversion  OutDataTypeStr=single  SaturateOnIntegerOverflow=off  RndMeth=Floor
  Cast2 : DataTypeConversion  OutDataTypeStr=single  SaturateOnIntegerOverflow=off  RndMeth=Floor
  Compare To Constant : simulink/Logic and Bit Operations/Compare To Constant  relop=<=  const=0  OutDataTypeStr=boolean
  Compare To Constant2 : simulink/Logic and Bit Operations/Compare To Constant  relop=<=  const=5  OutDataTypeStr=boolean
  Detect Rise Positive : simulink/Logic and Bit Operations/Detect Rise Positive  vinit=0  OutDataTypeStr=boolean
  Gain1 : Gain  Gain=1/3.6
  Gain3 : Gain  Gain=-1
  Gain4 : Gain  Gain=1/3.6
  I_Gain : Constant  Value=single(2)
  Integr_StartPoint : Constant  Value=single(0)
  Latch_on : Subsystem
  Logical Operator1 : Logic  AllPortsSameDT=off  OutDataTypeStr=boolean
  Logical Operator2 : Logic  Operator=NOT  AllPortsSameDT=off  OutDataTypeStr=boolean
  Logical Operator3 : Logic  Operator=OR  AllPortsSameDT=off  OutDataTypeStr=boolean
  Logical Operator4 : Logic  AllPortsSameDT=off  OutDataTypeStr=boolean
  Logical Operator5 : Logic  AllPortsSameDT=off  OutDataTypeStr=boolean
  OR : Logic  Operator=OR  AllPortsSameDT=off  OutDataTypeStr=boolean
  P_Gain : Constant  Value=single(20)
  Product : Product
  Product1 : Product
  Product2 : Product
  Relational Operator : RelationalOperator  Operator=<  OutDataTypeStr=boolean  RndMeth=Simplest  InputSameDT=off
  Relational Operator1 : RelationalOperator  Operator=<  OutDataTypeStr=boolean  RndMeth=Simplest  InputSameDT=off
  Relational Operator2 : RelationalOperator  OutDataTypeStr=boolean  RndMeth=Simplest  InputSameDT=off
  Relational Operator7 : RelationalOperator  Operator=<  OutDataTypeStr=boolean  RndMeth=Simplest  InputSameDT=off
  Relational Operator8 : RelationalOperator  Operator=>  OutDataTypeStr=boolean  RndMeth=Simplest  InputSameDT=off
  ResetDelay : Constant  Value=single(0.5)
  RisingTimer : Subsystem
  Saturation : Saturate  UpperLimit=40  LowerLimit=0
  Saturation Dynamic : simulink/Discontinuities/Saturation Dynamic  OutMin=[]  OutMax=[]  OutDataTypeStr=Inherit: Same as second input  OutDataType=fixdt(1, 16)  OutScaling=2^-10  DoSatur=off
  Saturation Dynamic1 : simulink/Discontinuities/Saturation Dynamic  OutMin=[]  OutMax=[]  OutDataTypeStr=Inherit: Same as second input  OutDataType=fixdt(1, 16)  OutScaling=2^-10  DoSatur=off
  Saturation Dynamic2 : simulink/Discontinuities/Saturation Dynamic  OutMin=[]  OutMax=[]  OutDataTypeStr=Inherit: Same as second input  OutDataType=fixdt(1, 16)  OutScaling=2^-10  DoSatur=off
  Saturation1 : Saturate  UpperLimit=50  LowerLimit=0
  Saturation2 : Saturate  UpperLimit=400  LowerLimit=-100
  Switch{,1..3,6..7} (6 alike) : Switch  Criteria=u2 ~= 0  SaturateOnIntegerOverflow=off  InputSameDT=off
  TCS_TrqRequest_Max2 : Constant  Value=single(235)
  TCS_TrqRequest_Min1 : Constant  Value=single(0)
  TCS_TrqRequest_Min2 : Constant  Value=single(0)
  Trq_IReset : Constant  Value=single(0)
  Trq_I_FF : Constant  Value=single(20)
  Unit Delay{,1..5} (6 alike) : UnitDelay  SampleTime=-1  HasFrameUpgradeWarning=on
  VehSpd_SlipTarget_mps : Lookup_n-D  NumberOfTableDimensions=1  BreakpointsForDimension1=[0 3 25 30]  Table=[0.3,0.3,2.5,2.5]  ExtrapMethod=Clip  InternalRulePriority=Speed  RndMeth=Simplest
  VehicleStableTarget_mps : Lookup_n-D  NumberOfTableDimensions=1  BreakpointsForDimension1=[0,3,25,30]  Table=[0.4,0.4,1.2,1.2]  ExtrapMethod=Clip  InternalRulePriority=Speed  RndMeth=Simplest
  VehicleStableTarget_mps1 : Lookup_n-D  NumberOfTableDimensions=1  BreakpointsForDimension1=[0,3,25,30]  Table=[0.4,0.4,1.2,1.2]  ExtrapMethod=Clip  InternalRulePriority=Speed  RndMeth=Simplest
  Verror : Constant  Value=single(0)
  Verror1 : Constant  Value=single(0)
  Verror_Reset : Constant  Value=single(0)
  Verror_Reset1 : Constant  Value=single(0)
  TCS_flgActv : Outport
  TCS_TrqRequestFinal_Nm : Outport  Port=2
  wires:
  TCS_TrqRequest_Max2/1 -> Saturation Dynamic1/1
  [TCS_Actv] -> Switch2/2
  [TrqRequst_Act_Nm] -> Switch7/1
  [VehSpd_Ref_mps] -> VehicleStableTarget_mps1/1, Add13/1
  Integr_StartPoint/1 -> Switch/3
  VehicleStableTarget_mps1/1 -> Add13/2
  [VehSpd_Ref_mps] -> Add5/1, VehicleStableTarget_mps/1
  [VehSpd_RA_mps] -> Add12/1
  [TCS_Actv] -> Switch6/2
  Gain4/1 -> Saturation1/1  "VehSpd_RA_mps"
  [TCS_Actv] -> Detect Rise Positive/1
  Saturation Dynamic1/1 -> Saturation Dynamic2/1
  Logical Operator3/1 -> Latch_on/2(Reset)  "TCS_ExitFinal"
  ResetDelay/1 -> RisingTimer/2(Timer)
  Latch_on/1(flg_TCSActv) -> TCS_flgActv/1, [TCS_Actv]  "TCS_flgActv"
  Unit Delay4/1 -> Relational Operator8/1
  WhlSpd_kph/1 -> Cast1/1
  Relational Operator1/1 -> Logical Operator5/1
  Product/1 -> [P_Portion], Add7/1  "P_out"
  Relational Operator7/1 -> Latch_on/1(Set), Logical Operator2/1  "TCS_Trigger"
  Switch/1 -> Add6/2  "Trq_I_Start"
  Trq_I_FF/1 -> Switch1/1
  Add13/1 -> Add12/2
  [TrqRequst_Act_Nm] -> Relational Operator2/2
  Add2/1 -> Saturation2/1
  TCS_TrqRequest_Min2/1 -> Saturation Dynamic1/3
  Add4/1 -> Switch/1
  [TCS_Inactive] -> Logical Operator3/2
  Add10/1 -> Relational Operator/1
  VehicleStableTarget_mps/1 -> Add5/2
  TrqRequst_Act_Nm/1 -> Cast2/1
  [P_Portion] -> Gain3/1
  Gain1/1 -> Saturation/1  "VehSpd_FA_mps"
  Saturation1/1 -> Add1/2, [VehSpd_RA_mps]
  Product1/1 -> Saturation Dynamic/2  "I_Portion"
  Logical Operator5/1 -> Unit Delay3/1, Switch7/2  "TCS_Inactive"
  Cal_DeltaV_mps1/1 -> Relational Operator8/2
  Add11/1 -> Saturation Dynamic/1
  Unit Delay3/1 -> [TCS_Inactive]
  Logical Operator1/1 -> RisingTimer/1(Set)
  [P_Portion] -> Add11/2
  Switch2/1 -> TCS_TrqRequestFinal_Nm/1, Unit Delay2/1  "TCS_TrqRequestFinal_Nm"
  [TCS_TrqReqstRaw_Nm] -> Compare To Constant2/1, Relational Operator2/1
  Switch1/1 -> Add6/3  "Trq_I_FF"
  [VehSpd_RA_mps] -> Add10/1
  Unit Delay/1 -> Switch3/3
  Logical Operator2/1 -> Logical Operator1/1
  Trq_IReset/1 -> Switch1/3
  Verror1/1 -> Relational Operator1/2
  Relational Operator2/1 -> OR/1  "a"
  Switch7/1 -> Switch2/3
  Add12/1 -> Relational Operator1/1
  [P_Portion] -> Unit Delay1/1
  Unit Delay1/1 -> Add4/2
  Verror/1 -> Relational Operator/2
  Saturation Dynamic2/1 -> Switch2/1  "TCS_TrqRequest"
  [TrqRequst_Act_Nm] -> Saturation Dynamic2/2
  [TrqRequst_Act_Nm] -> Add11/1
  I_Gain/1 -> Product1/2
  Switch6/1 -> Product/1, Add2/2  "Verror_mps"
  Add9/1 -> Add1/1  "whlref"
  VehSpd_SlipTarget_mps/1 -> Add9/1
  [TCS_TrqReqstRaw_Nm] -> Unit Delay4/1
  Add5/1 -> Add10/2
  Saturation2/1 -> Unit Delay/1, Add6/1
  Add1/1 -> Switch6/1, [Verr_mps], Unit Delay5/1, Product2/1  "Verror"
  Verror_Reset/1 -> Switch6/3
  TCS_TrqRequest_Min1/1 -> Saturation Dynamic2/3
  Add7/1 -> Saturation Dynamic1/2, [TCS_TrqReqstRaw_Nm]  "TCS_TrqReqst_Raw"
  [Verr_mps] -> Relational Operator7/1
  Cal_DeltaV_mps/1 -> Relational Operator7/2
  Add6/1 -> Product1/1
  Relational Operator8/1 -> Logical Operator1/2  "fSat_Actuators"
  Relational Operator/1 -> Logical Operator4/1
  Saturation/1 -> Add9/2, VehSpd_SlipTarget_mps/1, [VehSpd_Ref_mps]
  P_Gain/1 -> Product/2
  Detect Rise Positive/1 -> Switch/2
  [TCS_Actv] -> Logical Operator4/2
  Gain3/1 -> Saturation Dynamic/3
  Logical Operator4/1 -> Switch1/2  "flg_I_FF"
  VehSpd_kph/1 -> Cast/1
  RisingTimer/1(TCSExit) -> Logical Operator3/1
  Saturation Dynamic/1 -> Add7/2  "I_Out"
  Cast/1 -> Gain1/1
  Cast1/1 -> Gain4/1
  Cast2/1 -> Add4/1, [TrqRequst_Act_Nm]  "TrqRequst_Act_Nm"
  Unit Delay5/1 -> Product2/2
  Product2/1 -> Compare To Constant/1
  Switch3/1 -> Add2/1  "Verror_mps"
  Compare To Constant/1 -> [crosszore]
  [crosszore] -> Switch3/2
  Verror_Reset1/1 -> Switch3/1
  Unit Delay2/1 -> Switch7/3
  Compare To Constant2/1 -> OR/2
  OR/1 -> Logical Operator5/2

== system VDSE_2019b1/14-DOF VEHICLE MODEL/POWERTRAIN AND BRAKES/VCU/打滑判断/加速度差判断 ==
  note: 输出“1”代表判定有效
  <VxFL_mps> : Inport
  <VxFR_mps> : Inport  Port=2
  <VxRL_mps> : Inport  Port=3
  <VxRR_mps> : Inport  Port=4
  IMU_Ax_mpss : Inport  Port=5
  Abs{,1..3} (4 alike) : Abs  SaturateOnIntegerOverflow=off
  Add{,1..3} (4 alike) : Sum  Inputs=+-
  Add{4..7} (4 alike) : Sum  Inputs=-+
  Compare To Constant{,1..3} (4 alike) : simulink/Logic and Bit Operations/Compare To Constant  relop=<=  const=thr2  OutDataTypeStr=boolean
  Divide{,1..3} (4 alike) : Product  Inputs=*/
  Filter : Subsystem
  Filter1 : Subsystem
  Filter2 : Subsystem
  Filter3 : Subsystem
  Unit Delay{,1..3} (4 alike) : UnitDelay  SampleTime=-1  HasFrameUpgradeWarning=on
  steptime{,1..3} (4 alike) : Constant  Value=single(0.01)
  y : Outport
  y1 : Outport  Port=2
  y2 : Outport  Port=3
  y3 : Outport  Port=4
  wires:
  Compare To Constant/1 -> y/1
  Compare To Constant2/1 -> y2/1
  Abs2/1 -> Compare To Constant2/1
  Add1/1 -> Abs1/1
  Abs/1 -> Compare To Constant/1
  [IMU_Ax_mpss] -> Add3/2
  [IMU_Ax_mpss] -> Add2/2
  [IMU_Ax_mpss] -> Add/2
  Abs3/1 -> Compare To Constant3/1
  Compare To Constant3/1 -> y3/1
  Compare To Constant1/1 -> y1/1
  [IMU_Ax_mpss] -> Add1/2
  Add/1 -> Abs/1
  Add3/1 -> Abs3/1
  Abs1/1 -> Compare To Constant1/1
  Add2/1 -> Abs2/1
  <VxFL_mps>/1 -> Add4/2, Unit Delay/1
  Unit Delay/1 -> Add4/1
  Add4/1 -> Divide/1
  steptime/1 -> Divide/2
  Divide/1 -> Filter/1(In)
  IMU_Ax_mpss/1 -> [IMU_Ax_mpss]
  steptime1/1 -> Divide1/2
  Add5/1 -> Divide1/1
  Unit Delay1/1 -> Add5/1
  <VxFR_mps>/1 -> Unit Delay1/1, Add5/2
  Divide1/1 -> Filter1/1(In)
  steptime2/1 -> Divide2/2
  Add6/1 -> Divide2/1
  Unit Delay2/1 -> Add6/1
  <VxRL_mps>/1 -> Unit Delay2/1, Add6/2
  Divide2/1 -> Filter2/1(In)
  steptime3/1 -> Divide3/2
  Add7/1 -> Divide3/1
  Unit Delay3/1 -> Add7/1
  <VxRR_mps>/1 -> Unit Delay3/1, Add7/2
  Divide3/1 -> Filter3/1(In)
  Filter/1(Out) -> Add/1
  Filter1/1(Out) -> Add1/1
  Filter2/1(Out) -> Add2/1
  Filter3/1(Out) -> Add3/1

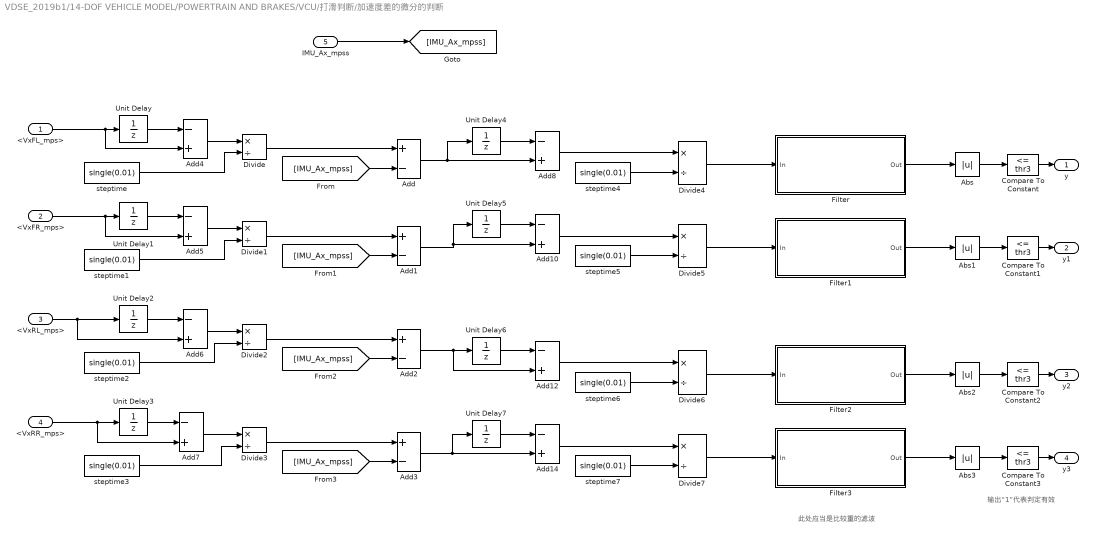
== system VDSE_2019b1/14-DOF VEHICLE MODEL/POWERTRAIN AND BRAKES/VCU/打滑判断/加速度差的微分的判断 ==
  note: 此处应当是比较重的滤波
  note: 输出“1”代表判定有效
  <VxFL_mps> : Inport
  <VxFR_mps> : Inport  Port=2
  <VxRL_mps> : Inport  Port=3
  <VxRR_mps> : Inport  Port=4
  IMU_Ax_mpss : Inport  Port=5
  Abs{,1..3} (4 alike) : Abs  SaturateOnIntegerOverflow=off
  Add{,1..3} (4 alike) : Sum  Inputs=+-
  Add{4..8,10,12,14} (8 alike) : Sum  Inputs=-+
  Compare To Constant{,1..3} (4 alike) : simulink/Logic and Bit Operations/Compare To Constant  relop=<=  const=thr3  OutDataTypeStr=boolean
  Divide{,1..7} (8 alike) : Product  Inputs=*/
  Filter : Subsystem
  Filter1 : Subsystem
  Filter2 : Subsystem
  Filter3 : Subsystem
  Unit Delay{,1..7} (8 alike) : UnitDelay  SampleTime=-1  HasFrameUpgradeWarning=on
  steptime{,1..7} (8 alike) : Constant  Value=single(0.01)
  y : Outport
  y1 : Outport  Port=2
  y2 : Outport  Port=3
  y3 : Outport  Port=4
  wires:
  Divide3/1 -> Add3/1
  <VxRR_mps>/1 -> Add7/2, Unit Delay3/1
  Unit Delay3/1 -> Add7/1
  Add7/1 -> Divide3/1
  steptime3/1 -> Divide3/2
  Divide2/1 -> Add2/1
  <VxRL_mps>/1 -> Add6/2, Unit Delay2/1
  Unit Delay2/1 -> Add6/1
  Add6/1 -> Divide2/1
  steptime2/1 -> Divide2/2
  Divide1/1 -> Add1/1
  <VxFR_mps>/1 -> Add5/2, Unit Delay1/1
  Unit Delay1/1 -> Add5/1
  Add5/1 -> Divide1/1
  steptime1/1 -> Divide1/2
  IMU_Ax_mpss/1 -> [IMU_Ax_mpss]
  Divide/1 -> Add/1
  steptime/1 -> Divide/2
  Add4/1 -> Divide/1
  Unit Delay/1 -> Add4/1
  <VxFL_mps>/1 -> Unit Delay/1, Add4/2
  Abs1/1 -> Compare To Constant1/1
  [IMU_Ax_mpss] -> Add1/2
  Compare To Constant1/1 -> y1/1
  Compare To Constant3/1 -> y3/1
  Abs3/1 -> Compare To Constant3/1
  [IMU_Ax_mpss] -> Add/2
  [IMU_Ax_mpss] -> Add2/2
  [IMU_Ax_mpss] -> Add3/2
  Abs/1 -> Compare To Constant/1
  Abs2/1 -> Compare To Constant2/1
  Compare To Constant2/1 -> y2/1
  Compare To Constant/1 -> y/1
  Add/1 -> Add8/2, Unit Delay4/1
  Unit Delay4/1 -> Add8/1
  Add8/1 -> Divide4/1
  steptime4/1 -> Divide4/2
  Divide4/1 -> Filter/1(In)
  steptime5/1 -> Divide5/2
  Add10/1 -> Divide5/1
  Unit Delay5/1 -> Add10/1
  Add1/1 -> Unit Delay5/1, Add10/2
  Divide5/1 -> Filter1/1(In)
  Divide6/1 -> Filter2/1(In)
  Add2/1 -> Add12/2, Unit Delay6/1
  Add12/1 -> Divide6/1
  steptime6/1 -> Divide6/2
  Unit Delay6/1 -> Add12/1
  steptime7/1 -> Divide7/2
  Add14/1 -> Divide7/1
  Add3/1 -> Unit Delay7/1, Add14/2
  Unit Delay7/1 -> Add14/1
  Divide7/1 -> Filter3/1(In)
  Filter/1(Out) -> Abs/1
  Filter1/1(Out) -> Abs1/1
  Filter2/1(Out) -> Abs2/1
  Filter3/1(Out) -> Abs3/1

== system VDSE_2019b1/14-DOF VEHICLE MODEL/POWERTRAIN AND BRAKES/VCU/打滑判断/速差判断 ==
  note: 输出“1”代表判定有效
  <VxFL_mps> : Inport
  <VxFR_mps> : Inport  Port=2
  <VxRL_mps> : Inport  Port=3
  <VxRR_mps> : Inport  Port=4
  VehSpd_mps : Inport  Port=5
  Abs{,1..3} (4 alike) : Abs  SaturateOnIntegerOverflow=off
  Add{,1..3} (4 alike) : Sum  Inputs=+-
  Compare To Constant{,1..3} (4 alike) : simulink/Logic and Bit Operations/Compare To Constant  relop=<=  const=thr1  OutDataTypeStr=boolean
  y : Outport
  y1 : Outport  Port=2
  y2 : Outport  Port=3
  y3 : Outport  Port=4
  wires:
  Add2/1 -> Abs2/1
  Abs1/1 -> Compare To Constant1/1
  <VxRR_mps>/1 -> Add3/1
  Add3/1 -> Abs3/1
  Add/1 -> Abs/1
  [VehSpd_mps] -> Add1/2
  <VxRL_mps>/1 -> Add2/1
  <VxFR_mps>/1 -> Add1/1
  Compare To Constant1/1 -> y1/1
  Compare To Constant3/1 -> y3/1
  Abs3/1 -> Compare To Constant3/1
  [VehSpd_mps] -> Add/2
  [VehSpd_mps] -> Add2/2
  [VehSpd_mps] -> Add3/2
  Abs/1 -> Compare To Constant/1
  Add1/1 -> Abs1/1
  Abs2/1 -> Compare To Constant2/1
  <VxFL_mps>/1 -> Add/1
  Compare To Constant2/1 -> y2/1
  Compare To Constant/1 -> y/1
  VehSpd_mps/1 -> [VehSpd_mps]

== system VDSE_2019b1/14-DOF VEHICLE MODEL/POWERTRAIN AND BRAKES/VCU/车速估计/Filter ==
  In : Inport
  Add : Sum
  Constant : Constant  Value=single(0)
  Constant1 : Constant  Value=single(100)
  Constant2 : Constant  Value=single(15)
  Constant3 : Constant  Value=single(-15)
  Gain : Gain  Gain=0
  Gain1 : Gain
  Rate Limiter Dynamic : simulink/Discontinuities/Rate Limiter Dynamic
  Saturation Dynamic : simulink/Discontinuities/Saturation Dynamic  OutMin=[]  OutMax=[]  OutDataTypeStr=Inherit: Same as second input  OutDataType=fixdt(1, 16)  OutScaling=2^-10  DoSatur=off
  Unit Delay : UnitDelay  SampleTime=-1  HasFrameUpgradeWarning=on
  VehVxEst_mps : Outport
  wires:
  In/1 -> Saturation Dynamic/2
  Saturation Dynamic/1 -> Rate Limiter Dynamic/2
  Constant1/1 -> Saturation Dynamic/1
  Constant/1 -> Saturation Dynamic/3
  Unit Delay/1 -> Gain/1
  Gain/1 -> Add/1
  Gain1/1 -> Add/2
  Rate Limiter Dynamic/1 -> Gain1/1, Unit Delay/1
  Add/1 -> VehVxEst_mps/1
  Constant2/1 -> Rate Limiter Dynamic/1
  Constant3/1 -> Rate Limiter Dynamic/3

== system VDSE_2019b1/14-DOF VEHICLE MODEL/POWERTRAIN AND BRAKES/VCU/车速估计/Filter1 ==
  In : Inport
  Add : Sum
  Constant : Constant  Value=single(-100)
  Constant1 : Constant  Value=single(100)
  Constant2 : Constant  Value=single(10)
  Constant3 : Constant  Value=single(-10)
  Gain : Gain  Gain=0.3
  Gain1 : Gain  Gain=0.7
  Rate Limiter Dynamic : simulink/Discontinuities/Rate Limiter Dynamic
  Saturation Dynamic : simulink/Discontinuities/Saturation Dynamic  OutMin=[]  OutMax=[]  OutDataTypeStr=Inherit: Same as second input  OutDataType=fixdt(1, 16)  OutScaling=2^-10  DoSatur=off
  Unit Delay : UnitDelay  SampleTime=-1  HasFrameUpgradeWarning=on
  Out : Outport
  wires:
  In/1 -> Saturation Dynamic/2
  Saturation Dynamic/1 -> Rate Limiter Dynamic/2
  Constant1/1 -> Saturation Dynamic/1
  Constant/1 -> Saturation Dynamic/3
  Constant2/1 -> Rate Limiter Dynamic/1
  Constant3/1 -> Rate Limiter Dynamic/3
  Unit Delay/1 -> Gain/1
  Gain/1 -> Add/1
  Add/1 -> Out/1
  Gain1/1 -> Add/2
  Rate Limiter Dynamic/1 -> Unit Delay/1, Gain1/1

== system VDSE_2019b1/14-DOF VEHICLE MODEL/POWERTRAIN AND BRAKES/VCU/车速估计/Subsystem ==
  <VxFL_mps> : Inport
  <VxFR_mps> : Inport  Port=2
  <VxRL_mps> : Inport  Port=3
  <VxRR_mps> : Inport  Port=4
  Add3 : Sum  Inputs=++++
  Add4 : Sum  Inputs=+--
  Gain1 : Gain  Gain=1/2
  Min3 : MinMax  Function=max  Inputs=4
  Min4 : MinMax  Inputs=4
  Subsystem : Subsystem  Commented=on
  MiddleWhlSpd_mps : Outport
  wires:
  Add4/1 -> Gain1/1
  Add3/1 -> Add4/1
  Min3/1 -> Add4/3
  <VxRR_mps>/1 -> Min3/4, Add3/1, Min4/4
  <VxRL_mps>/1 -> Min3/3, Min4/3, Add3/2
  <VxFR_mps>/1 -> Min4/2, Min3/2, Add3/3
  Min4/1 -> Add4/2
  <VxFL_mps>/1 -> Add3/4, Min4/1, Min3/1
  Gain1/1 -> MiddleWhlSpd_mps/1  "MaxWhlSpd_mps"

== system VDSE_2019b1/14-DOF VEHICLE MODEL/SUSPENSION/FRONT SUSPENSION/SUSPENSION FL/FL ==
  z [m] : Inport
  Vz [m/s] : Inport  Port=2
  phi [rad] : Inport  Port=3
  phi_dot [rad/s] : Inport  Port=4
  theta [rad] : Inport  Port=5
  theta_dot [rad/s] : Inport  Port=6
  zFR [m] : Inport  Port=7
  yFL_road [m] : Inport  Port=8
  Constant : Constant  Value=zFL_dot0
  Constant1 : Constant  Value=zFL0
  Constant10 : Constant  Value=ctF
  Constant2 : Constant  Value=cF
  Constant3 : Constant  Value=wF
  Constant4 : Constant  Value=lF
  Constant5 : Constant  Value=kF
  Constant6 : Constant  Value=kRF
  Constant7 : Constant  Value=ktF
  Constant8 : Constant  Value=mF
  Constant9 : Constant  Value=g
  Derivative : Derivative
  Integrator : Integrator  InitialConditionSource=external
  Integrator1 : Integrator  InitialConditionSource=external
  MATLAB Function : MATLAB Function  TreatAsAtomicUnit=on
  zFL [m] : Outport
  zFL_dot [m/s] : Outport  Port=2
  wires:
  Constant9/1 -> MATLAB Function/9(g)
  Constant8/1 -> MATLAB Function/1(mF)
  Constant7/1 -> MATLAB Function/5(ktF)
  Constant6/1 -> MATLAB Function/4(kRF)
  Constant5/1 -> MATLAB Function/3(kF)
  Constant4/1 -> MATLAB Function/8(lF)
  Constant3/1 -> MATLAB Function/7(wF)
  Constant2/1 -> MATLAB Function/2(cF)
  zFR [m]/1 -> MATLAB Function/18(zFR)
  theta_dot [rad/s]/1 -> MATLAB Function/17(theta_dot)
  theta [rad]/1 -> MATLAB Function/16(theta)
  phi [rad]/1 -> MATLAB Function/14(phi)
  z [m]/1 -> MATLAB Function/12(z)
  yFL_road [m]/1 -> Derivative/1, MATLAB Function/10(yFL_road)
  Integrator/1 -> zFL [m]/1, MATLAB Function/19(zFL)  "zFL"
  Integrator1/1 -> zFL_dot [m/s]/1, MATLAB Function/20(zFL_dot), Integrator/1  "zFL_dot"
  MATLAB Function/1(zFL_dot_dot) -> Integrator1/1  "zFL_dot_dot"
  Vz [m/s]/1 -> MATLAB Function/13(Vz)
  phi_dot [rad/s]/1 -> MATLAB Function/15(phi_dot)
  Constant/1 -> Integrator1/2
  Constant1/1 -> Integrator/2
  Constant10/1 -> MATLAB Function/6(ctF)
  Derivative/1 -> MATLAB Function/11(yFL_road_dot)
